simulink model "asyncip_sl_1_sm_ip_test"  (Simulink 7.8)
settings: Solver=ode4  SolverMode=SingleTasking  StartTime=0.0  StopTime=inf  FixedStep=5e-005  MaxStep=0.01  RelTol=1e-3  AbsTol=1e-6
undefined symbols (not defined in the file or in its folder): IP, UDP
libraries: opal_lib x2, rtlab x2, rtio_generic_ip x1
settings Model: Creator=jwu  LastModifiedBy=ACS  ExtModeTrigMode=oneshot  ExtModeArmWhenConnect=off  BufferReuse=off
settings DataIOCC: ExternalInput=[]  InitialState=[]  LimitDataPoints=off  SaveOutput=off  SaveTime=off  SignalLoggingName=sigsOut
settings OptimizationCC: BooleanDataType=off  OptimizeBlockIOStorage=off  BufferReuse=off  ExpressionFolding=off  FoldNonRolledExpr=off  LocalBlockOutputs=off  InitFltsAndDblsToZero=on
settings DebuggingCC: SaveWithParameterizedLinksMsg=none  SignalResolutionControl=TryResolveAllWithWarning  SolverPrmCheckMsg=none  InheritedTsInSrcMsg=none  MultiTaskDSMMsg=warning  MultiTaskCondExecSysMsg=none  FcnCallInpInsideContextMsg=Use local settings  StrictBusMsg=None
settings HardwareCC: TargetUnknown=on
settings RTWCC: GenCodeOnly=on  IncludeERTFirstTime=on
settings CodeAppCC: IgnoreCustomStorageClasses=off
settings GRTTargetCC: TargetFcnLib=ansi_tfl_tmw.mat

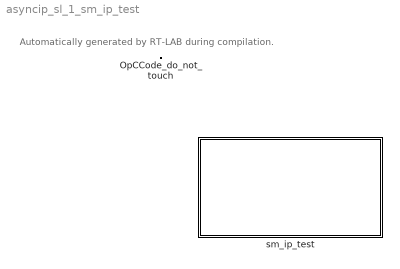
== system asyncip_sl_1_sm_ip_test ==
  note: Automatically generated by RT-LAB during compilation.
  OpCCode_do_not_touch : opal_lib/Communication/OpCCode  SystemSampleTime=-1
  sm_ip_test : Subsystem

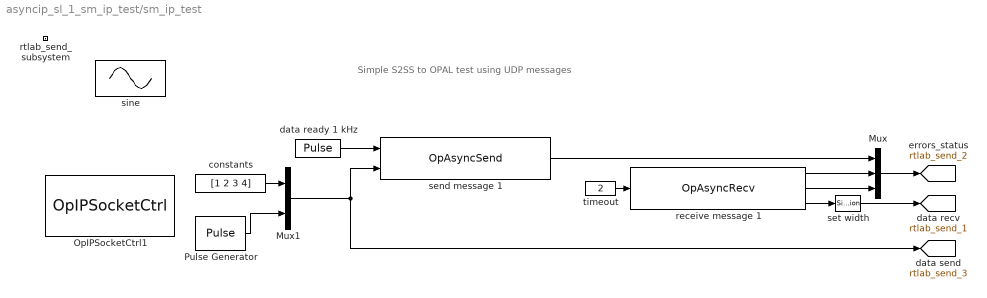
== system asyncip_sl_1_sm_ip_test/sm_ip_test ==
  note: Simple S2SS to OPAL test using UDP messages
  Mux : Mux  Inputs=3
  Mux1 : Mux  Inputs=2
  OpIPSocketCtrl1 : rtio_generic_ip/OpIPSocketCtrl  ctl_id=1  proto=UDP/IP  ip_addr_remote=137.226.160.91  ip_port_remote=10200  ip_port_local=10201  ip_addr_mcast=0.0.0.0  exe_name=AsyncIP
  Pulse Generator : DiscretePulseGenerator  PulseType=Time based  Amplitude=5  Period=0.1  PulseWidth=30
  constants : Constant  Value=[1 2 3 4]
  data ready 1 kHz : DiscretePulseGenerator  SampleTime=0.001
  receive message 1 : rtlab/Communication/Asynchronous/OpAsyncRecv  ctl_id=1  recv_id=1  enable_param=off  fp1=1  fp2=2  fp3=3  fp4=4  fp5=5  sp1=string1  sp2=string2  sp3=string3  sp4=string4  sp5=string5
  rtlab_send_subsystem : Subsystem  Priority=-100
      mask Display: text(0,0,'');
  send message 1 : rtlab/Communication/Asynchronous/OpAsyncSend  ctl_id=1  send_id=1  mode=DONT_NEED_REPLY  enable_param=off  fp1=1  fp2=2  fp3=3  fp4=4  fp5=5  sp1=string1  sp2=string2  sp3=string3  sp4=string4  sp5=string5
  set width : SignalSpecification  Dimensions=5
  sine : Sin  Amplitude=1.5  Frequency=50
  timeout : Constant  Value=2
  tag scope: rtlab_send_1=global, rtlab_send_2=global, rtlab_send_3=global
  wires:
  receive message 1/3 -> set width/1
  receive message 1/1 -> Mux/2
  receive message 1/2 -> Mux/3
  timeout/1 -> receive message 1/1
  send message 1/1 -> Mux/1
  Mux/1 -> [rtlab_send_2]
  set width/1 -> [rtlab_send_1]
  constants/1 -> Mux1/1
  Mux1/1 -> send message 1/2, [rtlab_send_3]
  data ready 1 kHz/1 -> send message 1/1
  Pulse Generator/1 -> Mux1/2

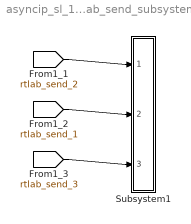
== system asyncip_sl_1_sm_ip_test/sm_ip_test/rtlab_send_subsystem ==
  Subsystem1 : Subsystem
  wires:
  [rtlab_send_2] -> Subsystem1/1(In1)
  [rtlab_send_1] -> Subsystem1/2(In2)
  [rtlab_send_3] -> Subsystem1/3(In3)

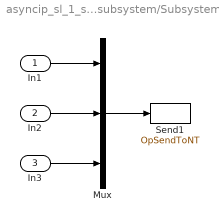
== system asyncip_sl_1_sm_ip_test/sm_ip_test/rtlab_send_subsystem/Subsystem1 ==
  In1 : Inport
  In2 : Inport  Port=2
  In3 : Inport  Port=3
  Mux : Mux  Inputs=3
  Send1 : opal_lib/Communication/OpSendToNT  Acqu_group=1
  wires:
  Mux/1 -> Send1/1
  In1/1 -> Mux/1
  In2/1 -> Mux/2
  In3/1 -> Mux/3
